simulink model "cosim_fir"  (R2015b)
settings: Solver=FixedStepDiscrete  SolverMode=SingleTasking  StartTime=0.0  StopTime=10.0  RelTol=1e-3
libraries: simulink x1
settings Model: Creator=at-mt  LastModifiedBy=amatsumo
settings DataIOCC: SaveFormat=Array  SignalLoggingSaveFormat=ModelDataLogs  SaveOutput=off  SignalLogging=off  SaveTime=off
settings OptimizationCC: BlockReduction=off  ConditionallyExecuteInputs=off  DefaultParameterBehavior=Inlined  ExpressionDepthLimit=2147483647
settings DebuggingCC: AlgebraicLoopMsg=error  UnderspecifiedInitializationDetection=Classic  MergeDetectMultiDrivingBlocksExec=none  SolverPrmCheckMsg=warning  InheritedTsInSrcMsg=none  SingleTaskRateTransMsg=error  ParameterPrecisionLossMsg=none  ParameterTunabilityLossMsg=none  FcnCallInpInsideContextMsg=UseLocalSettings  StateNameClashWarn=warning
settings HardwareCC: ProdBitPerPointer=32  ProdLargestAtomicFloat=None  ProdIntDivRoundTo=Undefined  ProdEndianess=Unspecified  ProdWordSize=32  ProdHWDeviceType=ASIC/FPGA->ASIC/FPGA  ProdEqTarget=off
settings GRTTargetCC: GeneratePreprocessorConditionals=Disable all  CombineOutputUpdateFcns=off  GRTInterface=on
settings ConfigComp: CovModelRefEnable=Off  CovSFcnEnable=off

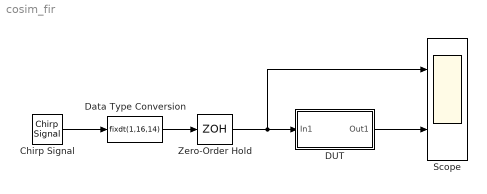
== system cosim_fir ==
  Chirp Signal : simulink/Sources/Chirp Signal  f1=10  T=10  f2=500
  DUT : Subsystem
  Data Type Conversion : DataTypeConversion  OutDataTypeStr=fixdt(1,16,14)  RndMeth=Nearest
  Scope : Scope  NumInputPorts=2
  Zero-Order Hold : ZeroOrderHold  SampleTime=1/1000
  wires:
  Chirp Signal/1 -> Data Type Conversion/1
  Zero-Order Hold/1 -> DUT/1(In1), Scope/1
  Data Type Conversion/1 -> Zero-Order Hold/1
  DUT/1(Out1) -> Scope/2

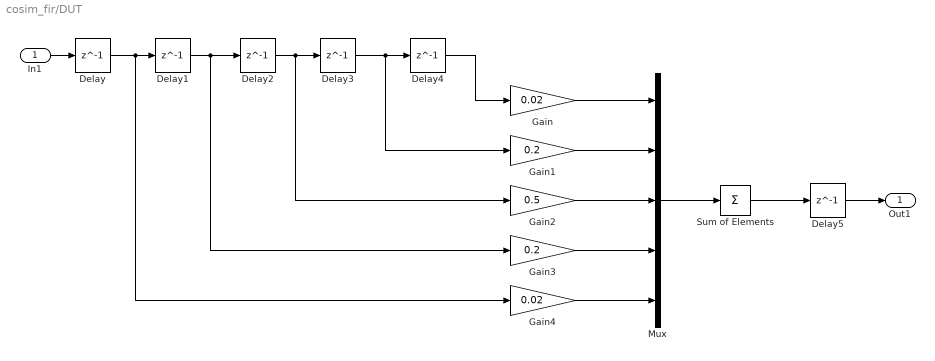
== system cosim_fir/DUT ==
  In1 : Inport
  Delay{,1..5} (6 alike) : Delay  DelayLength=1
  Gain : Gain  Gain=0.02  OutDataTypeStr=Inherit: Same as input
  Gain1 : Gain  Gain=0.2  OutDataTypeStr=Inherit: Same as input
  Gain2 : Gain  Gain=0.5  OutDataTypeStr=Inherit: Same as input
  Gain3 : Gain  Gain=0.2  OutDataTypeStr=Inherit: Same as input
  Gain4 : Gain  Gain=0.02  OutDataTypeStr=Inherit: Same as input
  Mux : Mux  Inputs=5
  Sum of Elements : Sum  Inputs=+
  Out1 : Outport
  wires:
  Sum of Elements/1 -> Delay5/1
  Gain4/1 -> Mux/5
  Gain3/1 -> Mux/4
  Gain2/1 -> Mux/3
  Gain1/1 -> Mux/2
  Gain/1 -> Mux/1
  Mux/1 -> Sum of Elements/1
  In1/1 -> Delay/1
  Delay5/1 -> Out1/1
  Delay1/1 -> Delay2/1, Gain3/1
  Delay2/1 -> Delay3/1, Gain2/1
  Delay3/1 -> Delay4/1, Gain1/1
  Delay4/1 -> Gain/1
  Delay/1 -> Delay1/1, Gain4/1
